simulink model "Symmetry_Inverter_imagined"  (Simulink 8.1)
settings: Solver=ode23t  StartTime=0.0  StopTime=tfin  RelTol=1e-4
values from neighbouring files (symbols this model uses):
  amp_feedback_saturation = 400    [Symmetry_ini_COPY.m]
  Butterworth_filter_order = 8    [Symmetry_ini_COPY.m]
  Capacitive_Load_R_RC = [60e-3,  120e-3,  80e-3;                                 3e-3, 15e-3, 9e-3]    [Symmetry_ini_COPY.m]
  initial_value = [0.00,0.00,0.00,                  0,0,0]    [Symmetry_ini_COPY.m]
  k_symmetrcal_gain = 1e2    (= 100)    [Symmetry_ini_COPY.m]
  L_Source = [3.185e-3, 3.185e-3, 3.185e-3]    [Symmetry_ini_COPY.m]
  Load_R = [50,50,50]    [Symmetry_ini_COPY.m]
  Load_RL = [35.35,   35.35,   35.35;                   0.1125,  0.1125,  0.1125]    [Symmetry_ini_COPY.m]
  Network_Wire_Resistance = 0.4    [Symmetry_ini_COPY.m]
  NetworkBreaker = [1e5,1e5,1e5,1e5]    [Symmetry_ini_COPY.m]
  P_gain = 1e-4    (= 0.0001)    [Symmetry_ini_COPY.m]
  phase_feedback_saturation = pi    (= 3.14159265359)    [Symmetry_ini_COPY.m]
  Phase_Source = [0,-2/3*pi,-4/3*pi]    [Symmetry_ini_COPY.m]
  PowerGain = [1e-5,1e-5,0]    [Symmetry_ini_COPY.m]
  PV_Power_Capacity = 2e4    (= 20000)    [Symmetry_ini_COPY.m]
  R_Source = [0.4, 0.4, 0.4]    [Symmetry_ini_COPY.m]
  sample = 10e-5    (= 0.0001)    [Symmetry_ini_COPY.m]    (also in animated_norms.m; save_data.m)
  Source_Frequency = [50,50,50]    [Symmetry_ini_COPY.m]
  Start_Control = 1    [Symmetry_ini_COPY.m]
  START_Load_R = [0.001,100,100]    [Symmetry_ini_COPY.m]
  START_Load_RC = [100,100,0.001]    [Symmetry_ini_COPY.m]
  START_Load_RL = [100,0.001,100]    [Symmetry_ini_COPY.m]
  step_size = [1,1,1,                  0.08,0.08,0.08]    [Symmetry_ini_COPY.m]
  test_step = [0.5,0.5,0.5,                  0.02,0.02,0.02]    [Symmetry_ini_COPY.m]
  TransformerBreaker = [1e5,1e5,1e5;                     1e5,1e5,1e5]    [Symmetry_ini_COPY.m]
  Urms_Source = [230,230,230]    [Symmetry_ini_COPY.m]
libraries: powerlib x105, simulink x18, dspsigops x10, commsequence2 x6, powerlib_extras x6, dspxfrm3 x3, dsparch4 x3
(part 2 of 2)

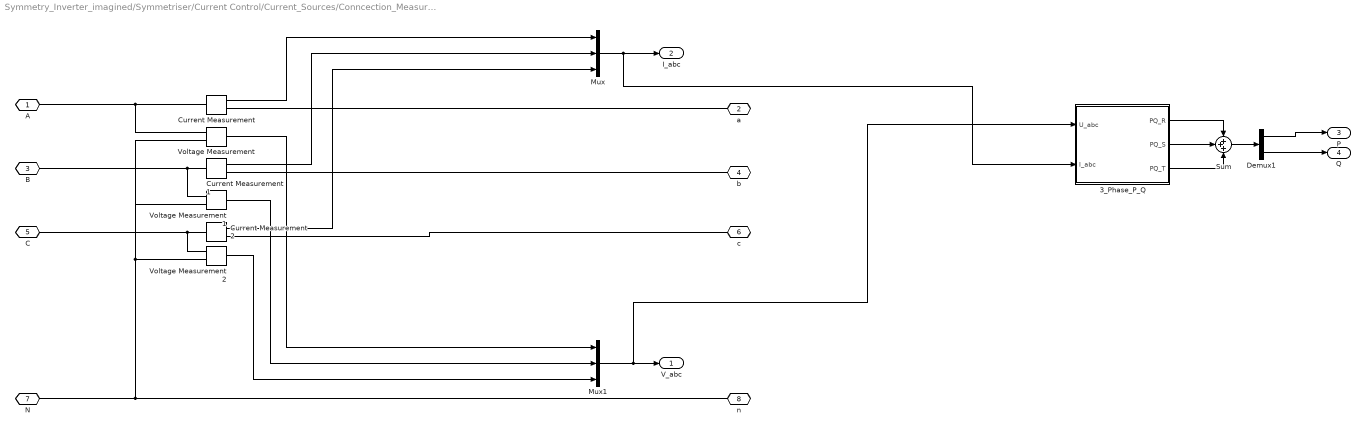
== system Symmetry_Inverter_imagined/Symmetriser/Current Control/Current_Sources/Conncection_Measurements ==
  3_Phase_P_Q : Subsystem
  Current Measurement : powerlib/Measurements/Current Measurement  PhasorSimulation=off  OutputType=Complex  PSBequivalent=0
  Current Measurement1 : powerlib/Measurements/Current Measurement  PhasorSimulation=off  OutputType=Complex  PSBequivalent=0
  Current Measurement2 : powerlib/Measurements/Current Measurement  PhasorSimulation=off  OutputType=Complex  PSBequivalent=0
  Demux1 : Demux  Outputs=2
  Mux : Mux  Inputs=3
  Mux1 : Mux  Inputs=3
  Sum : Sum  Inputs=+++
  Voltage Measurement : powerlib/Measurements/Voltage Measurement  PhasorSimulation=off  OutputType=Complex  PSBequivalent=0
  Voltage Measurement1 : powerlib/Measurements/Voltage Measurement  PhasorSimulation=off  OutputType=Complex  PSBequivalent=0
  Voltage Measurement2 : powerlib/Measurements/Voltage Measurement  PhasorSimulation=off  OutputType=Complex  PSBequivalent=0
  A : PMIOPort  Port=1  Side=Left
  a : PMIOPort  Port=2  Side=Right
  B : PMIOPort  Port=3  Side=Left
  b : PMIOPort  Port=4  Side=Right
  C : PMIOPort  Port=5  Side=Left
  c : PMIOPort  Port=6  Side=Right
  N : PMIOPort  Port=7  Side=Left
  n : PMIOPort  Port=8  Side=Right
  V_abc : Outport
  I_abc : Outport  Port=2
  P : Outport  Port=3
  Q : Outport  Port=4
  wires:
  Current Measurement1/1 -> Mux/2
  Current Measurement/1 -> Mux/1
  Voltage Measurement/1 -> Mux1/1
  Current Measurement2/1 -> Mux/3
  Voltage Measurement1/1 -> Mux1/2
  Voltage Measurement2/1 -> Mux1/3
  3_Phase_P_Q/2(PQ_S) -> Sum/2
  3_Phase_P_Q/1(PQ_R) -> Sum/1
  3_Phase_P_Q/3(PQ_T) -> Sum/3
  Mux/1 -> 3_Phase_P_Q/2(I_abc), I_abc/1
  Mux1/1 -> 3_Phase_P_Q/1(U_abc), V_abc/1
  Sum/1 -> Demux1/1
  Demux1/1 -> P/1
  Demux1/2 -> Q/1
  connections:
  Current Measurement2/RConn1 -- c/RConn1
  Current Measurement/RConn1 -- a/RConn1
  Current Measurement1/RConn1 -- b/RConn1
  Voltage Measurement2/LConn1 -- C/RConn1 -- Current Measurement2/LConn1
  Voltage Measurement2/LConn2 -- Voltage Measurement1/LConn2 -- Voltage Measurement/LConn2 -- N/RConn1 -- n/RConn1
  Voltage Measurement1/LConn1 -- B/RConn1 -- Current Measurement1/LConn1
  Voltage Measurement/LConn1 -- A/RConn1 -- Current Measurement/LConn1

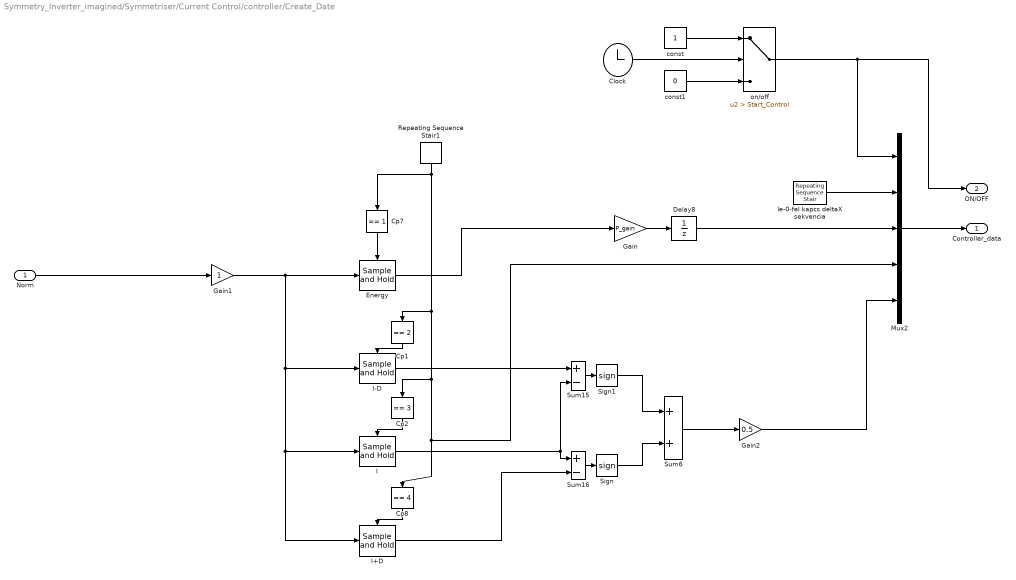
== system Symmetry_Inverter_imagined/Symmetriser/Current Control/controller/Create_Date ==
  Norm : Inport
  Clock : Clock
      settings: Decimation=CLK
  Cp1 : simulink/Logic and Bit Operations/Compare To Constant  relop===  const=2  OutDataTypeStr=uint8  ZeroCross=off
  Cp2 : simulink/Logic and Bit Operations/Compare To Constant  relop===  const=3  OutDataTypeStr=uint8  ZeroCross=off
  Cp7 : simulink/Logic and Bit Operations/Compare To Constant  relop===  const=1  OutDataTypeStr=uint8  ZeroCross=off
  Cp8 : simulink/Logic and Bit Operations/Compare To Constant  relop===  const=4  OutDataTypeStr=uint8  ZeroCross=off
  Delay8 : UnitDelay  SampleTime=0.02
  Energy : dspsigops/Sample and Hold  trig=Rising edge  initCond=18  latchinput=off
  Gain : Gain  Gain=P_gain
  Gain1 : Gain
  Gain2 : Gain  Gain=0.5
  I : dspsigops/Sample and Hold  trig=Rising edge  initCond=0  latchinput=off
  I+D : dspsigops/Sample and Hold  trig=Rising edge  initCond=0  latchinput=off
  I-D : dspsigops/Sample and Hold  trig=Rising edge  initCond=0  latchinput=off
  Mux2 : Mux  Inputs=5
  Repeating Sequence Stair1 : simulink/Sources/Repeating Sequence Stair  OutValues=[1 2 3 4 5].'  tsamp=stair_sample  OutMin=[]  OutMax=[]  OutDataTypeStr=float('double')  OutputDataTypeScalingMode=Specify via dialog  OutDataType=float('double')  ConRadixGroup=Best Precision: Vector-wise  OutScaling=2^-12
  Sign : Signum
  Sign1 : Signum
  Sum15 : Sum  Inputs=+-
  Sum16 : Sum  Inputs=+-
  Sum6 : Sum
  const : Constant
  const1 : Constant  Value=0
  le-0-fel kapcs deltaX sekvencia : simulink/Sources/Repeating Sequence Stair  OutValues=[-1 0 1 0 0].'  tsamp=switch_sample  OutMin=[]  OutMax=[]  OutDataTypeStr=float('double')  OutputDataTypeScalingMode=Specify via dialog  OutDataType=float('double')  ConRadixGroup=Best Precision: Vector-wise  OutScaling=2^-12
  on/off : Switch  Criteria=u2 > Threshold  Threshold=Start_Control
  Controller_data : Outport
  ON/OFF : Outport  Port=2
  wires:
  Cp1/1 -> I-D/Trigger
  Repeating Sequence Stair1/1 -> Cp7/1, Mux2/4, Cp8/1, Cp2/1, Cp1/1
  Cp7/1 -> Energy/Trigger
  Energy/1 -> Gain/1
  Cp2/1 -> I/Trigger
  Cp8/1 -> I+D/Trigger
  Gain1/1 -> I+D/1, I/1, I-D/1, Energy/1
  I-D/1 -> Sum15/1
  I/1 -> Sum15/2, Sum16/1
  I+D/1 -> Sum16/2
  Sum16/1 -> Sign/1
  Sum15/1 -> Sign1/1
  Gain/1 -> Delay8/1
  Sign/1 -> Sum6/2
  Sign1/1 -> Sum6/1
  le-0-fel kapcs deltaX sekvencia/1 -> Mux2/2
  Delay8/1 -> Mux2/3
  on/off/1 -> Mux2/1, ON/OFF/1
  Mux2/1 -> Controller_data/1
  Norm/1 -> Gain1/1
  Sum6/1 -> Gain2/1
  const/1 -> on/off/1
  const1/1 -> on/off/3
  Clock/1 -> on/off/2
  Gain2/1 -> Mux2/5

== system Symmetry_Inverter_imagined/Symmetriser/Current Control/controller/Phase_control_S ==
  Control : Inport
  Cp3 : simulink/Logic and Bit Operations/Compare To Constant  relop===  const=5  OutDataTypeStr=uint8  ZeroCross=off
  Delay : UnitDelay  SampleTime=0.001
  Delay4 : UnitDelay  SampleTime=0.02
  Demux2 : Demux  Outputs=5
  I Controller : dspsigops/Sample and Hold  trig=Rising edge  initCond=0  latchinput=off
  I3 Step : Constant  Value=step_size(5)
  "I3 init " : Constant  Value=initial_value(5)
  I3 test step : Constant  Value=test_step(5)
  Mask : simulink/Sources/Repeating Sequence Stair  OutValues=[0 0 0 0 1 0].'  tsamp=mask_sample  OutMin=[]  OutMax=[]  OutDataTypeStr=float('double')  OutputDataTypeScalingMode=Specify via dialog  OutDataType=float('double')  ConRadixGroup=Best Precision: Vector-wise  OutScaling=2^-12
  Product : Product  RndMeth=Zero
  Product12 : Product  RndMeth=Zero
  Product4 : Product  Inputs=4  RndMeth=Zero
  Product8 : Product  Inputs=4  RndMeth=Zero
  Saturation : Saturate  UpperLimit=phase_feedback_saturation  LowerLimit=-phase_feedback_saturation
  Sum : Sum  Inputs=|++
  Sum5 : Sum  Inputs=+++
  phase_S : Outport
  wires:
  Control/1 -> Demux2/1
  Product12/1 -> phase_S/1
  Product8/1 -> Sum/1
  Delay/1 -> Saturation/1
  "I3 init "/1 -> Sum5/2
  Delay4/1 -> Sum5/3
  Demux2/5 -> Product8/2
  Demux2/4 -> Product/2
  Demux2/3 -> Product4/3, Product8/1
  Demux2/2 -> Product4/2
  Demux2/1 -> Product12/1, Product8/4
  I3 Step/1 -> Product8/3
  Cp3/1 -> I Controller/Trigger
  Mask/1 -> Product/1, Product4/4
  Sum5/1 -> Product12/2
  I3 test step/1 -> Product4/1
  I Controller/1 -> Delay4/1, Delay/1
  Product4/1 -> Sum5/1
  Product/1 -> Cp3/1
  Sum/1 -> I Controller/1
  Saturation/1 -> Sum/2

== system Symmetry_Inverter_imagined/Symmetriser/Current Control/controller/amp_control_R ==
  Control : Inport
  k : Inport  Port=2
  Cp3 : simulink/Logic and Bit Operations/Compare To Constant  relop===  const=5  OutDataTypeStr=uint8  ZeroCross=off
  Delay : UnitDelay  SampleTime=0.001
  Delay4 : UnitDelay  SampleTime=0.02
  Demux2 : Demux  Outputs=5
  I Controller : dspsigops/Sample and Hold  trig=Rising edge  initCond=0  latchinput=off
  I3 Step : Constant  Value=step_size(1)
  "I3 init " : Constant  Value=initial_value(1)
  I3 test step : Constant  Value=test_step(1)
  Mask : simulink/Sources/Repeating Sequence Stair  OutValues=[1 0 0 0 0 0].'  tsamp=mask_sample  OutMin=[]  OutMax=[]  OutDataTypeStr=float('double')  OutputDataTypeScalingMode=Specify via dialog  OutDataType=float('double')  ConRadixGroup=Best Precision: Vector-wise  OutScaling=2^-12
  Product : Product  RndMeth=Zero
  Product12 : Product  RndMeth=Zero
  Product4 : Product  Inputs=4  RndMeth=Zero
  Product8 : Product  Inputs=5  RndMeth=Zero
  Saturation : Saturate  UpperLimit=amp_feedback_saturation  LowerLimit=-amp_feedback_saturation
  Sum : Sum  Inputs=|++
  Sum5 : Sum  Inputs=+++
  amp_R : Outport
  wires:
  Control/1 -> Demux2/1
  Product12/1 -> amp_R/1
  Product8/1 -> Sum/1
  Delay/1 -> Saturation/1
  "I3 init "/1 -> Sum5/2
  Delay4/1 -> Sum5/3
  Demux2/5 -> Product8/2
  Demux2/4 -> Product/2
  Demux2/3 -> Product4/3, Product8/1
  Demux2/2 -> Product4/2
  Demux2/1 -> Product12/1, Product8/4
  I3 Step/1 -> Product8/3
  Cp3/1 -> I Controller/Trigger
  Mask/1 -> Product/1, Product4/4
  Sum5/1 -> Product12/2
  I3 test step/1 -> Product4/1
  I Controller/1 -> Delay4/1, Delay/1
  Product4/1 -> Sum5/1
  Product/1 -> Cp3/1
  Sum/1 -> I Controller/1
  Saturation/1 -> Sum/2
  k/1 -> Product8/5

== system Symmetry_Inverter_imagined/Symmetriser/Current Control/controller/amp_control_S ==
  Control : Inport
  k : Inport  Port=2
  Cp3 : simulink/Logic and Bit Operations/Compare To Constant  relop===  const=5  OutDataTypeStr=uint8  ZeroCross=off
  Delay : UnitDelay  SampleTime=0.001
  Delay4 : UnitDelay  SampleTime=0.02
  Demux2 : Demux  Outputs=5
  I Controller : dspsigops/Sample and Hold  trig=Rising edge  initCond=0  latchinput=off
  I3 Step : Constant  Value=step_size(2)
  "I3 init " : Constant  Value=initial_value(2)
  I3 test step : Constant  Value=test_step(2)
  Mask : simulink/Sources/Repeating Sequence Stair  OutValues=[0 1 0 0 0 0].'  tsamp=mask_sample  OutMin=[]  OutMax=[]  OutDataTypeStr=float('double')  OutputDataTypeScalingMode=Specify via dialog  OutDataType=float('double')  ConRadixGroup=Best Precision: Vector-wise  OutScaling=2^-12
  Product : Product  RndMeth=Zero
  Product12 : Product  RndMeth=Zero
  Product4 : Product  Inputs=4  RndMeth=Zero
  Product8 : Product  Inputs=5  RndMeth=Zero
  Saturation : Saturate  UpperLimit=amp_feedback_saturation  LowerLimit=-amp_feedback_saturation
  Sum : Sum  Inputs=|++
  Sum5 : Sum  Inputs=+++
  amp_S : Outport
  wires:
  Saturation/1 -> Sum/2
  Sum/1 -> I Controller/1
  Product/1 -> Cp3/1
  Product4/1 -> Sum5/1
  I Controller/1 -> Delay/1, Delay4/1
  I3 test step/1 -> Product4/1
  Sum5/1 -> Product12/2
  Mask/1 -> Product4/4, Product/1
  Cp3/1 -> I Controller/Trigger
  I3 Step/1 -> Product8/3
  Demux2/1 -> Product8/4, Product12/1
  Demux2/2 -> Product4/2
  Demux2/3 -> Product8/1, Product4/3
  Demux2/4 -> Product/2
  Demux2/5 -> Product8/2
  Delay4/1 -> Sum5/3
  "I3 init "/1 -> Sum5/2
  Delay/1 -> Saturation/1
  Product8/1 -> Sum/1
  Product12/1 -> amp_S/1
  Control/1 -> Demux2/1
  k/1 -> Product8/5

== system Symmetry_Inverter_imagined/Symmetriser/Current Control/controller/amp_control_T ==
  Control : Inport
  k : Inport  Port=2
  Cp3 : simulink/Logic and Bit Operations/Compare To Constant  relop===  const=5  OutDataTypeStr=uint8  ZeroCross=off
  Delay : UnitDelay  SampleTime=0.001
  Delay4 : UnitDelay  SampleTime=0.02
  Demux2 : Demux  Outputs=5
  I Controller : dspsigops/Sample and Hold  trig=Rising edge  initCond=0  latchinput=off
  I3 Step : Constant  Value=step_size(3)
  "I3 init " : Constant  Value=initial_value(3)
  I3 test step : Constant  Value=test_step(3)
  Mask : simulink/Sources/Repeating Sequence Stair  OutValues=[0 0 1 0 0 0].'  tsamp=mask_sample  OutMin=[]  OutMax=[]  OutDataTypeStr=float('double')  OutputDataTypeScalingMode=Specify via dialog  OutDataType=float('double')  ConRadixGroup=Best Precision: Vector-wise  OutScaling=2^-12
  Product : Product  RndMeth=Zero
  Product12 : Product  RndMeth=Zero
  Product4 : Product  Inputs=4  RndMeth=Zero
  Product8 : Product  Inputs=5  RndMeth=Zero
  Saturation : Saturate  UpperLimit=amp_feedback_saturation  LowerLimit=-amp_feedback_saturation
  Sum : Sum  Inputs=|++
  Sum5 : Sum  Inputs=+++
  amp_T : Outport
  wires:
  Control/1 -> Demux2/1
  Product12/1 -> amp_T/1
  Product8/1 -> Sum/1
  Delay/1 -> Saturation/1
  "I3 init "/1 -> Sum5/2
  Delay4/1 -> Sum5/3
  Demux2/5 -> Product8/2
  Demux2/4 -> Product/2
  Demux2/3 -> Product4/3, Product8/1
  Demux2/2 -> Product4/2
  Demux2/1 -> Product12/1, Product8/4
  I3 Step/1 -> Product8/3
  Cp3/1 -> I Controller/Trigger
  Mask/1 -> Product/1, Product4/4
  Sum5/1 -> Product12/2
  I3 test step/1 -> Product4/1
  I Controller/1 -> Delay4/1, Delay/1
  Product4/1 -> Sum5/1
  Product/1 -> Cp3/1
  Sum/1 -> I Controller/1
  Saturation/1 -> Sum/2
  k/1 -> Product8/5

== system Symmetry_Inverter_imagined/Symmetriser/Current Control/controller/phase_control_R ==
  Control : Inport
  Cp3 : simulink/Logic and Bit Operations/Compare To Constant  relop===  const=5  OutDataTypeStr=uint8  ZeroCross=off
  Delay : UnitDelay  SampleTime=0.001
  Delay4 : UnitDelay  SampleTime=0.02
  Demux2 : Demux  Outputs=5
  I Controller : dspsigops/Sample and Hold  trig=Rising edge  initCond=0  latchinput=off
  I3 Step : Constant  Value=step_size(4)
  "I3 init " : Constant  Value=initial_value(4)
  I3 test step : Constant  Value=test_step(4)
  Mask : simulink/Sources/Repeating Sequence Stair  OutValues=[0 0 0 1 0 0].'  tsamp=mask_sample  OutMin=[]  OutMax=[]  OutDataTypeStr=float('double')  OutputDataTypeScalingMode=Specify via dialog  OutDataType=float('double')  ConRadixGroup=Best Precision: Vector-wise  OutScaling=2^-12
  Product : Product  RndMeth=Zero
  Product12 : Product  RndMeth=Zero
  Product4 : Product  Inputs=4  RndMeth=Zero
  Product8 : Product  Inputs=4  RndMeth=Zero
  Saturation : Saturate  UpperLimit=phase_feedback_saturation  LowerLimit=-phase_feedback_saturation
  Sum : Sum  Inputs=|++
  Sum5 : Sum  Inputs=+++
  phase_R : Outport
  wires:
  Saturation/1 -> Sum/2
  Sum/1 -> I Controller/1
  Product/1 -> Cp3/1
  Product4/1 -> Sum5/1
  I Controller/1 -> Delay/1, Delay4/1
  I3 test step/1 -> Product4/1
  Sum5/1 -> Product12/2
  Mask/1 -> Product4/4, Product/1
  Cp3/1 -> I Controller/Trigger
  I3 Step/1 -> Product8/3
  Demux2/1 -> Product12/1, Product8/4
  Demux2/2 -> Product4/2
  Demux2/3 -> Product8/1, Product4/3
  Demux2/4 -> Product/2
  Demux2/5 -> Product8/2
  Delay4/1 -> Sum5/3
  "I3 init "/1 -> Sum5/2
  Delay/1 -> Saturation/1
  Product8/1 -> Sum/1
  Product12/1 -> phase_R/1
  Control/1 -> Demux2/1

== system Symmetry_Inverter_imagined/Symmetriser/Current Control/controller/phase_control_T ==
  Control : Inport
  Cp3 : simulink/Logic and Bit Operations/Compare To Constant  relop===  const=5  OutDataTypeStr=uint8  ZeroCross=off
  Delay : UnitDelay  SampleTime=0.001
  Delay4 : UnitDelay  SampleTime=0.02
  Demux2 : Demux  Outputs=5
  I Controller : dspsigops/Sample and Hold  trig=Rising edge  initCond=0  latchinput=off
  I3 Step : Constant  Value=step_size(6)
  "I3 init " : Constant  Value=initial_value(6)
  I3 test step : Constant  Value=test_step(6)
  Mask : simulink/Sources/Repeating Sequence Stair  OutValues=[0 0 0 0 0 1].'  tsamp=mask_sample  OutMin=[]  OutMax=[]  OutDataTypeStr=float('double')  OutputDataTypeScalingMode=Specify via dialog  OutDataType=float('double')  ConRadixGroup=Best Precision: Vector-wise  OutScaling=2^-12
  Product : Product  RndMeth=Zero
  Product12 : Product  RndMeth=Zero
  Product4 : Product  Inputs=4  RndMeth=Zero
  Product8 : Product  Inputs=4  RndMeth=Zero
  Saturation : Saturate  UpperLimit=phase_feedback_saturation  LowerLimit=-phase_feedback_saturation
  Sum : Sum  Inputs=|++
  Sum5 : Sum  Inputs=+++
  phase_S : Outport
  wires:
  Saturation/1 -> Sum/2
  Sum/1 -> I Controller/1
  Product/1 -> Cp3/1
  Product4/1 -> Sum5/1
  I Controller/1 -> Delay/1, Delay4/1
  I3 test step/1 -> Product4/1
  Sum5/1 -> Product12/2
  Mask/1 -> Product4/4, Product/1
  Cp3/1 -> I Controller/Trigger
  I3 Step/1 -> Product8/3
  Demux2/1 -> Product12/1, Product8/4
  Demux2/2 -> Product4/2
  Demux2/3 -> Product8/1, Product4/3
  Demux2/4 -> Product/2
  Demux2/5 -> Product8/2
  Delay4/1 -> Sum5/3
  "I3 init "/1 -> Sum5/2
  Delay/1 -> Saturation/1
  Product8/1 -> Sum/1
  Product12/1 -> phase_S/1
  Control/1 -> Demux2/1

== system Symmetry_Inverter_imagined/Symmetriser/Current Control/Current_Sources/Conncection_Measurements/3_Phase_P_Q ==
  U_abc : Inport
  I_abc : Inport  Port=2
  Demux1 : Demux  Outputs=3
  Demux3 : Demux  Outputs=3
  P Q in3 : powerlib_extras/Measurements/Active & Reactive Power  f1=Source_Frequency(1)
  P Q in4 : powerlib_extras/Measurements/Active & Reactive Power  f1=Source_Frequency(2)
  P Q in5 : powerlib_extras/Measurements/Active & Reactive Power  f1=Source_Frequency(3)
  PQ_R : Outport
  PQ_S : Outport  Port=2
  PQ_T : Outport  Port=3
  wires:
  P Q in3/1 -> PQ_R/1
  P Q in4/1 -> PQ_S/1
  P Q in5/1 -> PQ_T/1
  Demux3/1 -> P Q in3/1
  Demux3/2 -> P Q in4/1
  Demux3/3 -> P Q in5/1
  Demux1/1 -> P Q in3/2
  Demux1/2 -> P Q in4/2
  Demux1/3 -> P Q in5/2
  U_abc/1 -> Demux3/1
  I_abc/1 -> Demux1/1

== matlab function Symmetriser/Calculate_Norms/Mearusement_calc/geometrial norm ==
  data: amplitude_R input double; GEO_norm output double; amplitude_S input double; amplitude_T input double; phase_R input double; phase_S input double; phase_T input double
function GEO_norm = fcn(amplitude_R,amplitude_S,amplitude_T,phase_R,phase_S,phase_T)
%#codegen

x1=[0,0,0,0];
y1=[0,0,0,0];
x2=[0,0,0,0];
y2=[0,0,0,0];

GEO_norm=0;

coder.extrinsic('geometry_solver')

        %% Ideal parameters
        Amplitude_1=[325.3,325.3,325.3];                     %[V]
        %Phase_1=[-1.5855,2.6033,0.5089];
        Phase_1=[0,-2/3*pi,-4/3*pi];                     %[rad]
      
        %% Real parameters
        Amplitude_2=[amplitude_R,amplitude_S,amplitude_T];
        Phase_2=[phase_R,phase_S,phase_T];
        %Extension of the vectors with the first element to get closed triangles on
        %plots and for use as polygons
        Amplitude_1_ex=[Amplitude_1 Amplitude_1(1)];
        Phase_1_ex=[Phase_1 Phase_1(1)];
        Amplitude_2_ex=[Amplitude_2 Amplitude_2(1)];
        Phase_2_ex=[Phase_2 Phase_2(1)];
        
        GEO_norm=geometry_solver(Amplitude_1_ex, Phase_1_ex, Amplitude_2_ex, Phase_2_ex);

== matlab function Symmetriser/Current Control/controller/MATLAB Function1 ==
  data: amp input double; CC output double; phase input double; t input double
function CC = fcn(amp,phase,t)
%#codegen

CC = zeros(3,1);
CC_mtx=[amp(1),50,phase(1),0;...
        amp(1),50,phase(1)-2/3*pi,0;...
        amp(1),50,phase(1)-4/3*pi,0];
% T=1;
% CC=[(CC_mtx(1,1)*sin(2*pi*CC_mtx(1,2)*t+CC_mtx(1,3))+CC_mtx(1,4)).*(1-exp(-t/T)),...
%     (CC_mtx(2,1)*sin(2*pi*CC_mtx(2,2)*t+CC_mtx(2,3))+CC_mtx(2,4)).*(1-exp(-t/T)),...
%     (CC_mtx(3,1)*sin(2*pi*CC_mtx(3,2)*t+CC_mtx(3,3))+CC_mtx(3,4)).*(1-exp(-t/T))]';

CC=[(CC_mtx(1,1)*sin(2*pi*CC_mtx(1,2)*t+CC_mtx(1,3))+CC_mtx(1,4)),...
    (CC_mtx(2,1)*sin(2*pi*CC_mtx(2,2)*t+CC_mtx(2,3))+CC_mtx(2,4)),...
    (CC_mtx(3,1)*sin(2*pi*CC_mtx(3,2)*t+CC_mtx(3,3))+CC_mtx(3,4))]';

== matlab function Symmetriser/Current Control/controller/MATLAB Function ==
  data: amp input double; CC output double; phase input double; t input double
function CC = fcn(amp,phase,t)
%#codegen
CC = zeros(3,1);

CC_mtx=[amp(1),50,phase(1),0;...
        amp(2),50,phase(2),0;...
        amp(3),50,phase(3),0];
% T=1;
% CC=[(CC_mtx(1,1)*sin(2*pi*CC_mtx(1,2)*t+CC_mtx(1,3))+CC_mtx(1,4)).*(1-exp(-t/T)),...
%     (CC_mtx(2,1)*sin(2*pi*CC_mtx(2,2)*t+CC_mtx(2,3))+CC_mtx(2,4)).*(1-exp(-t/T)),...
%     (CC_mtx(3,1)*sin(2*pi*CC_mtx(3,2)*t+CC_mtx(3,3))+CC_mtx(3,4)).*(1-exp(-t/T))]';

CC=[(CC_mtx(1,1)*sin(2*pi*CC_mtx(1,2)*t+CC_mtx(1,3))+CC_mtx(1,4)),...
    (CC_mtx(2,1)*sin(2*pi*CC_mtx(2,2)*t+CC_mtx(2,3))+CC_mtx(2,4)),...
    (CC_mtx(3,1)*sin(2*pi*CC_mtx(3,2)*t+CC_mtx(3,3))+CC_mtx(3,4))]';
